simulink model "Ground_rover_model"  (R2014b)
settings: Solver=ode45  StartTime=0.0  StopTime=10.0  RelTol=1e-3
settings Model: Creator=Samy.Amin  LastModifiedBy=Samy.Amin

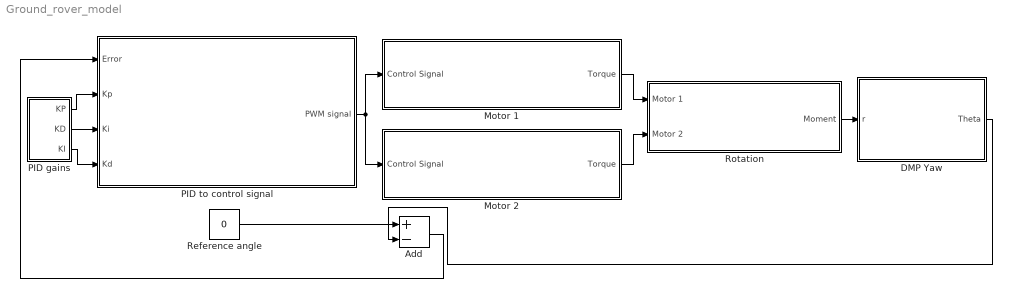
== system Ground_rover_model ==
  Add : Sum  Inputs=+-
  DMP Yaw : Subsystem
  Motor 1 : Subsystem
  Motor 2 : Subsystem
  PID gains : Subsystem
  "PID to control signal " : Subsystem
  Reference angle : Constant  Value=0
  Rotation : Subsystem
  wires:
  Rotation/1(Moment) -> DMP Yaw/1(r)
  "PID to control signal "/1("PWM signal ") -> Motor 2/1(Control Signal), Motor 1/1(Control Signal)
  Motor 1/1(Torque) -> Rotation/1(Motor 1)
  Motor 2/1(Torque) -> Rotation/2(Motor 2)
  DMP Yaw/1(Theta) -> Add/2
  PID gains/1(KP) -> "PID to control signal "/2(Kp)
  PID gains/2(KD) -> "PID to control signal "/3(Ki)
  PID gains/3(KI) -> "PID to control signal "/4(Kd)
  Reference angle/1 -> Add/1
  Add/1 -> "PID to control signal "/1(Error)

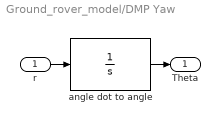
== system Ground_rover_model/DMP Yaw ==
  r : Inport
  angle dot to angle : TransferFcn  Denominator=[1 0]
  Theta : Outport
  wires:
  r/1 -> angle dot to angle/1
  angle dot to angle/1 -> Theta/1

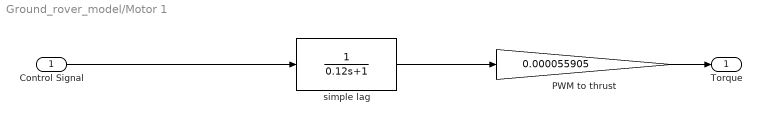
== system Ground_rover_model/Motor 1 ==
  Control Signal : Inport
  PWM to thrust : Gain  Gain=0.000055905
  simple lag : TransferFcn  Denominator=[0.12 1]
  Torque : Outport
  wires:
  Control Signal/1 -> simple lag/1
  simple lag/1 -> PWM to thrust/1
  PWM to thrust/1 -> Torque/1

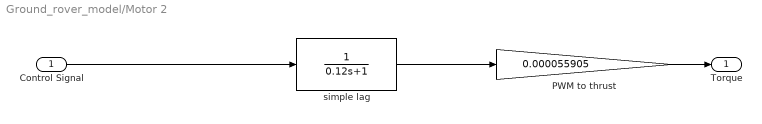
== system Ground_rover_model/Motor 2 ==
  Control Signal : Inport
  PWM to thrust : Gain  Gain=0.000055905
  simple lag : TransferFcn  Denominator=[0.12 1]
  Torque : Outport
  wires:
  PWM to thrust/1 -> Torque/1
  simple lag/1 -> PWM to thrust/1
  Control Signal/1 -> simple lag/1

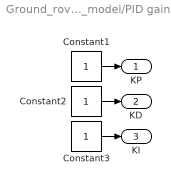
== system Ground_rover_model/PID gains ==
  Constant1 : Constant
  Constant2 : Constant
  Constant3 : Constant
  KP : Outport
  KD : Outport  Port=2
  KI : Outport  Port=3
  wires:
  Constant2/1 -> KD/1
  Constant3/1 -> KI/1
  Constant1/1 -> KP/1

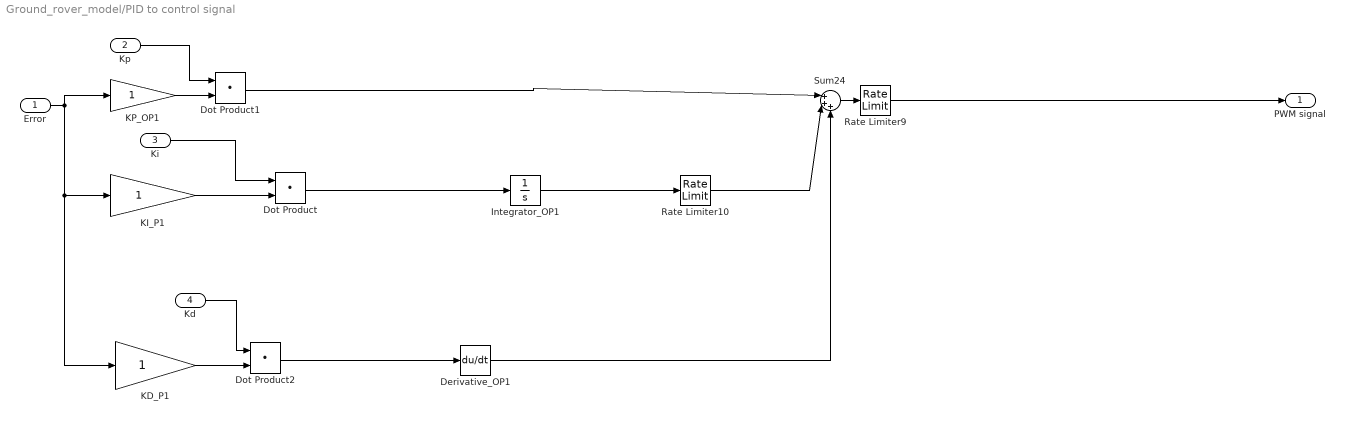
== system Ground_rover_model/PID to control signal  ==
  Error : Inport
  Kp : Inport  Port=2
  Ki : Inport  Port=3
  Kd : Inport  Port=4
  Derivative_OP1 : Derivative
  Dot Product : DotProduct  InputSameDT=on  OutDataTypeStr=Inherit: Inherit via internal rule
  Dot Product1 : DotProduct  InputSameDT=on  OutDataTypeStr=Inherit: Inherit via internal rule
  Dot Product2 : DotProduct  InputSameDT=on  OutDataTypeStr=Inherit: Inherit via internal rule
  Integrator_OP1 : Integrator
  KD_P1 : Gain
  KI_P1 : Gain
  KP_OP1 : Gain
  Rate Limiter10 : RateLimiter  RisingSlewLimit=399  FallingSlewLimit=-399  SampleTimeMode=inherited
  Rate Limiter9 : RateLimiter  RisingSlewLimit=551  FallingSlewLimit=-551  SampleTimeMode=inherited
  Sum24 : Sum  Inputs=|+++
  "PWM signal " : Outport
  wires:
  Rate Limiter10/1 -> Sum24/2
  Error/1 -> KD_P1/1, KI_P1/1, KP_OP1/1
  Derivative_OP1/1 -> Sum24/3
  Integrator_OP1/1 -> Rate Limiter10/1
  Rate Limiter9/1 -> "PWM signal "/1
  Sum24/1 -> Rate Limiter9/1
  Kp/1 -> Dot Product1/1
  KP_OP1/1 -> Dot Product1/2
  Dot Product1/1 -> Sum24/1
  Ki/1 -> Dot Product/1
  KI_P1/1 -> Dot Product/2
  Dot Product/1 -> Integrator_OP1/1
  Kd/1 -> Dot Product2/1
  KD_P1/1 -> Dot Product2/2
  Dot Product2/1 -> Derivative_OP1/1

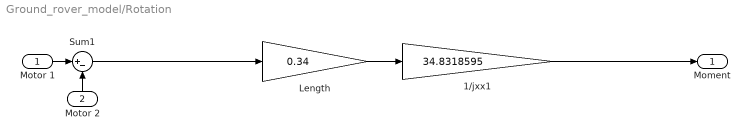
== system Ground_rover_model/Rotation ==
  Motor 1 : Inport
  Motor 2 : Inport  Port=2
  1/jxx1 : Gain  Gain=34.8318595
  Length : Gain  Gain=0.34
  Sum1 : Sum  Inputs=|+-
  Moment : Outport
  wires:
  Sum1/1 -> Length/1
  Motor 1/1 -> Sum1/1
  Motor 2/1 -> Sum1/2
  1/jxx1/1 -> Moment/1
  Length/1 -> 1/jxx1/1
